simulink model "Taller5_Desarollo"  (R2024a)
settings: Solver=VariableStepAuto  StartTime=0.0  StopTime=0.05  RelTol=1e-3
undefined symbols (not defined in the file): den, num
settings Model: Creator=geova  LastModifiedBy=geova

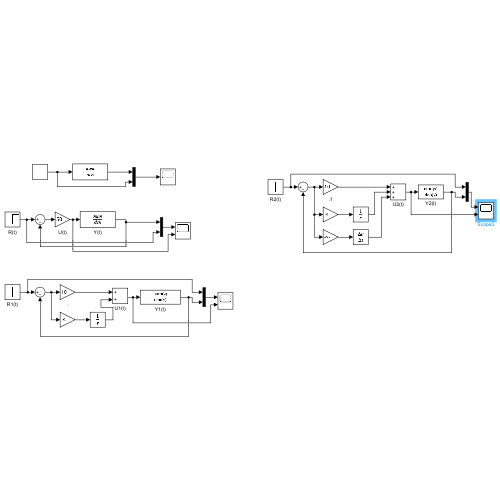
[thumbnail: Simulink's stored preview of the top-level diagram]
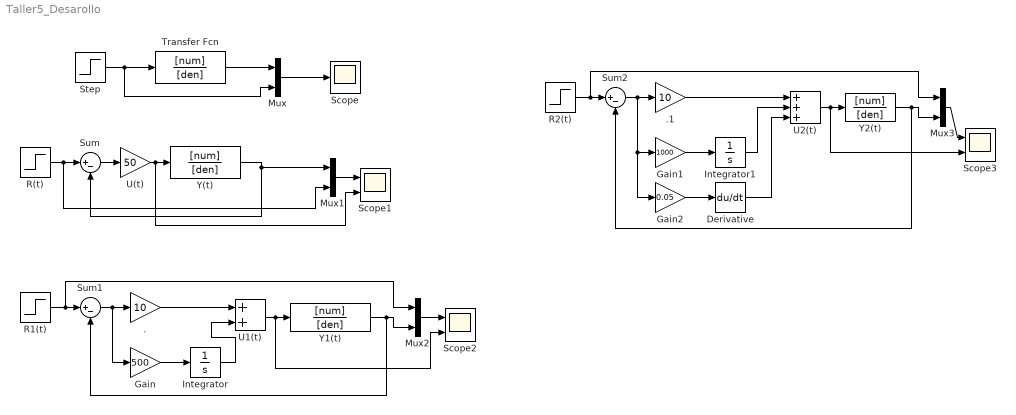
== system Taller5_Desarollo ==
  . : Gain  Gain=10
  .1 : Gain  Gain=10
  Derivative : Derivative
  Gain : Gain  Gain=500
  Gain1 : Gain  Gain=1000
  Gain2 : Gain  Gain=0.05
  Integrator : Integrator
  Integrator1 : Integrator
  Mux{,1..3} (4 alike) : Mux  Inputs=2
  R(t) : Step  Time=10*10^(-3)  After=5  SampleTime=0.0001
  R1(t) : Step  Time=10*10^(-3)  After=5  SampleTime=0.0001
  R2(t) : Step  Time=10*10^(-3)  After=5  SampleTime=0.0001
  Scope : Scope
  Scope1 : Scope  NumInputPorts=2
  Scope2 : Scope  NumInputPorts=2
  Scope3 : Scope  NumInputPorts=2
  Step : Step  Time=10*10^(-3)  After=5  SampleTime=0.0001
  Sum : Sum  Inputs=|+-
  Sum1 : Sum  Inputs=|+-
  Sum2 : Sum  Inputs=|+-
  Transfer Fcn : TransferFcn  Numerator=[num]  Denominator=[den]
  U(t) : Gain  Gain=50
  U1(t) : Sum
  U2(t) : Sum  Inputs=+++
  Y(t) : TransferFcn  Numerator=[num]  Denominator=[den]
  Y1(t) : TransferFcn  Numerator=[num]  Denominator=[den]
  Y2(t) : TransferFcn  Numerator=[num]  Denominator=[den]
  wires:
  Step/1 -> Mux/2, Transfer Fcn/1
  Transfer Fcn/1 -> Mux/1
  Mux/1 -> Scope/1
  Y(t)/1 -> Mux1/1, Sum/2
  U(t)/1 -> Scope1/2, Y(t)/1
  R(t)/1 -> Mux1/2, Sum/1
  Sum/1 -> U(t)/1
  Mux1/1 -> Scope1/1
  Sum1/1 -> Gain/1, ./1
  R1(t)/1 -> Mux2/1, Sum1/1
  Mux2/1 -> Scope2/1
  ./1 -> U1(t)/1
  U1(t)/1 -> Scope2/2, Y1(t)/1
  Y1(t)/1 -> Sum1/2, Mux2/2
  Integrator/1 -> U1(t)/2
  Gain/1 -> Integrator/1
  R2(t)/1 -> Mux3/1, Sum2/1
  Y2(t)/1 -> Sum2/2, Mux3/2
  Mux3/1 -> Scope3/1
  .1/1 -> U2(t)/1
  U2(t)/1 -> Scope3/2, Y2(t)/1
  Sum2/1 -> Gain2/1, Gain1/1, .1/1
  Gain1/1 -> Integrator1/1
  Integrator1/1 -> U2(t)/2
  Gain2/1 -> Derivative/1
  Derivative/1 -> U2(t)/3
